simulink model "nonLinearSim"  (R2021b)
settings: Solver=VariableStepAuto  StartTime=0.0  StopTime=50  MaxStep=0.01  RelTol=1e-3
undefined symbols (not defined in the file or in its folder): IRL, P, PE, SE
settings Model: Creator=rushik  LastModifiedBy=rushik
settings DataIOCC: SaveOutput=off  DSMLogging=off  SaveTime=off  ReturnWorkspaceOutputs=off

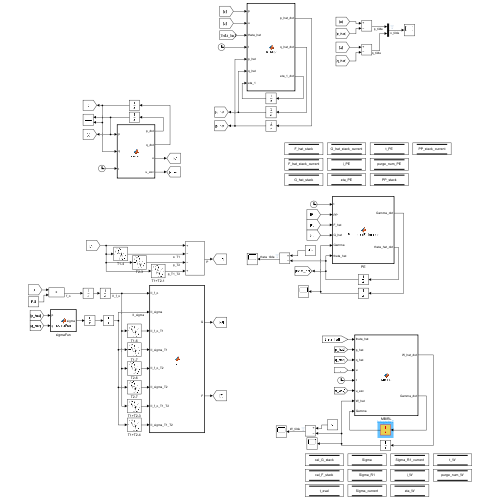
[thumbnail: Simulink's stored preview of the top-level diagram]
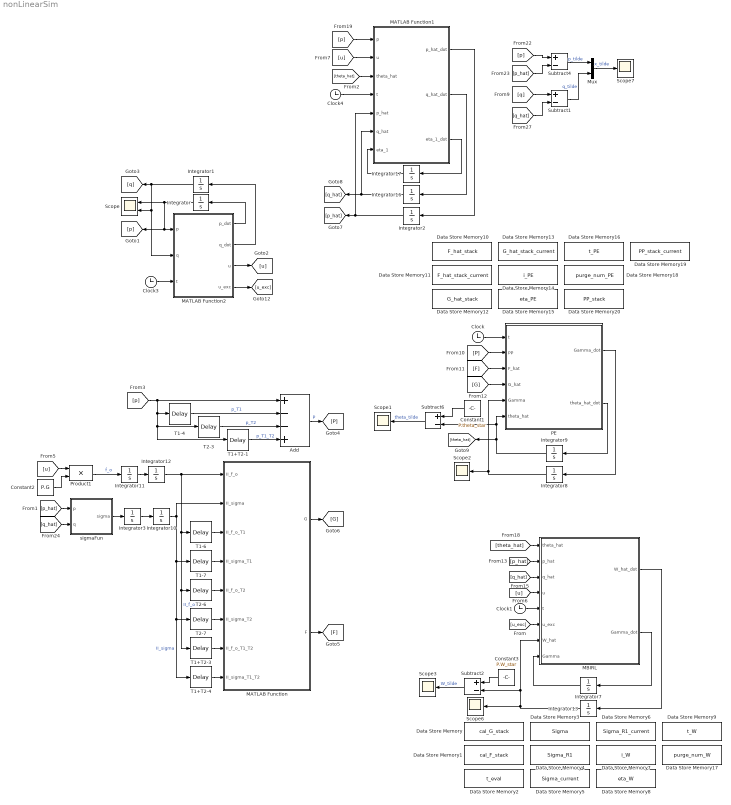
== system nonLinearSim ==
  Add : Sum  Inputs=+--+
  Clock{,1,3..4} (4 alike) : Clock
  Constant1 : Constant  Value=P.theta_star
  Constant2 : Constant  Value=P.G
  Constant3 : Constant  Value=P.W_star  VectorParams1D=off
  Data Store Memory : DataStoreMemory  DataStoreName=cal_G_stack  ReadBeforeWriteMsg=warning  WriteAfterWriteMsg=warning  WriteAfterReadMsg=warning  InitialValue=zeros(2*P.n^2,P.n*PE.N)  VectorParams1D=off  ShowAdditionalParam=off  OutDataTypeStr=double
  Data Store Memory1 : DataStoreMemory  DataStoreName=cal_F_stack  ReadBeforeWriteMsg=warning  WriteAfterWriteMsg=warning  WriteAfterReadMsg=warning  InitialValue=zeros(P.n,PE.N)  VectorParams1D=off  ShowAdditionalParam=off  OutDataTypeStr=double
  Data Store Memory10 : DataStoreMemory  DataStoreName=F_hat_stack  ReadBeforeWriteMsg=warning  WriteAfterWriteMsg=warning  WriteAfterReadMsg=warning  InitialValue=zeros(P.n,PE.N)  VectorParams1D=off  ShowAdditionalParam=off  OutDataTypeStr=double
  Data Store Memory11 : DataStoreMemory  DataStoreName=F_hat_stack_current  ReadBeforeWriteMsg=warning  WriteAfterWriteMsg=warning  WriteAfterReadMsg=warning  InitialValue=zeros(P.n,PE.N)  VectorParams1D=off  ShowAdditionalParam=off  OutDataTypeStr=double
  Data Store Memory12 : DataStoreMemory  DataStoreName=G_hat_stack  ReadBeforeWriteMsg=warning  WriteAfterWriteMsg=warning  WriteAfterReadMsg=warning  InitialValue=zeros(PE.L,PE.N)  VectorParams1D=off  ShowAdditionalParam=off  OutDataTypeStr=double
  Data Store Memory13 : DataStoreMemory  DataStoreName=G_hat_stack_current  ReadBeforeWriteMsg=warning  WriteAfterWriteMsg=warning  WriteAfterReadMsg=warning  InitialValue=zeros(PE.L,PE.N)  VectorParams1D=off  ShowAdditionalParam=off  OutDataTypeStr=double
  Data Store Memory14 : DataStoreMemory  DataStoreName=i_PE  ReadBeforeWriteMsg=warning  WriteAfterWriteMsg=warning  WriteAfterReadMsg=warning  InitialValue=1  VectorParams1D=off  ShowAdditionalParam=off  OutDataTypeStr=double
  Data Store Memory15 : DataStoreMemory  DataStoreName=eta_PE  ReadBeforeWriteMsg=warning  WriteAfterWriteMsg=warning  WriteAfterReadMsg=warning  VectorParams1D=off  ShowAdditionalParam=off  OutDataTypeStr=double
  Data Store Memory16 : DataStoreMemory  DataStoreName=t_PE  ReadBeforeWriteMsg=warning  WriteAfterWriteMsg=warning  WriteAfterReadMsg=warning  VectorParams1D=off  ShowAdditionalParam=off  OutDataTypeStr=double
  Data Store Memory17 : DataStoreMemory  DataStoreName=purge_num_W  ReadBeforeWriteMsg=warning  WriteAfterWriteMsg=warning  WriteAfterReadMsg=warning  VectorParams1D=off  ShowAdditionalParam=off  OutDataTypeStr=double
  Data Store Memory18 : DataStoreMemory  DataStoreName=purge_num_PE  ReadBeforeWriteMsg=warning  WriteAfterWriteMsg=warning  WriteAfterReadMsg=warning  VectorParams1D=off  ShowAdditionalParam=off  OutDataTypeStr=double
  Data Store Memory19 : DataStoreMemory  DataStoreName=PP_stack_current  ReadBeforeWriteMsg=warning  WriteAfterWriteMsg=warning  WriteAfterReadMsg=warning  InitialValue=zeros(P.n,PE.N)  VectorParams1D=off  ShowAdditionalParam=off  OutDataTypeStr=double
  Data Store Memory2 : DataStoreMemory  DataStoreName=t_eval  ReadBeforeWriteMsg=warning  WriteAfterWriteMsg=warning  WriteAfterReadMsg=warning  VectorParams1D=off  ShowAdditionalParam=off  OutDataTypeStr=double
  Data Store Memory20 : DataStoreMemory  DataStoreName=PP_stack  ReadBeforeWriteMsg=warning  WriteAfterWriteMsg=warning  WriteAfterReadMsg=warning  InitialValue=zeros(P.n,PE.N)  VectorParams1D=off  ShowAdditionalParam=off  OutDataTypeStr=double
  Data Store Memory3 : DataStoreMemory  DataStoreName=Sigma  ReadBeforeWriteMsg=warning  WriteAfterWriteMsg=warning  WriteAfterReadMsg=warning  InitialValue=zeros(2*IRL.N,IRL.num_weights)  VectorParams1D=off  ShowAdditionalParam=off  OutDataTypeStr=double
  Data Store Memory4 : DataStoreMemory  DataStoreName=Sigma_R1  ReadBeforeWriteMsg=warning  WriteAfterWriteMsg=warning  WriteAfterReadMsg=warning  InitialValue=zeros(2*IRL.N,1)  VectorParams1D=off  ShowAdditionalParam=off  OutDataTypeStr=double
  Data Store Memory5 : DataStoreMemory  DataStoreName=Sigma_current  ReadBeforeWriteMsg=warning  WriteAfterWriteMsg=warning  WriteAfterReadMsg=warning  InitialValue=zeros(2*IRL.N,IRL.num_weights)  VectorParams1D=off  ShowAdditionalParam=off  OutDataTypeStr=double
  Data Store Memory6 : DataStoreMemory  DataStoreName=Sigma_R1_current  ReadBeforeWriteMsg=warning  WriteAfterWriteMsg=warning  WriteAfterReadMsg=warning  InitialValue=zeros(2*IRL.N,1)  VectorParams1D=off  ShowAdditionalParam=off  OutDataTypeStr=double
  Data Store Memory7 : DataStoreMemory  DataStoreName=i_W  ReadBeforeWriteMsg=warning  WriteAfterWriteMsg=warning  WriteAfterReadMsg=warning  InitialValue=1  VectorParams1D=off  ShowAdditionalParam=off  OutDataTypeStr=double
  Data Store Memory8 : DataStoreMemory  DataStoreName=eta_W  ReadBeforeWriteMsg=warning  WriteAfterWriteMsg=warning  WriteAfterReadMsg=warning  VectorParams1D=off  ShowAdditionalParam=off  OutDataTypeStr=double
  Data Store Memory9 : DataStoreMemory  DataStoreName=t_W  ReadBeforeWriteMsg=warning  WriteAfterWriteMsg=warning  WriteAfterReadMsg=warning  VectorParams1D=off  ShowAdditionalParam=off  OutDataTypeStr=double
  Integrator : Integrator  InitialCondition=P.p_0
  Integrator1 : Integrator  InitialCondition=P.q_0
  Integrator10 : Integrator  InitialCondition=zeros(PE.L,1)
  Integrator11 : Integrator  InitialCondition=zeros(P.n,1)
  Integrator12 : Integrator  InitialCondition=zeros(P.n,1)
  Integrator13 : Integrator  InitialCondition=IRL.W_hat_0
  Integrator16 : Integrator  InitialCondition=SE.q_hat_0
  Integrator17 : Integrator
  Integrator2 : Integrator  InitialCondition=P.p_0
  Integrator3 : Integrator  InitialCondition=zeros(PE.L,1)
  Integrator7 : Integrator  InitialCondition=IRL.Gamma_W_0
  Integrator8 : Integrator  InitialCondition=PE.Gamma_0
  Integrator9 : Integrator  InitialCondition=PE.theta_hat_0
  MATLAB Function : MATLAB Function  TreatAsAtomicUnit=on
  MATLAB Function1 : MATLAB Function  TreatAsAtomicUnit=on
  MATLAB Function2 : MATLAB Function  TreatAsAtomicUnit=on
  MBIRL : MATLAB Function  TreatAsAtomicUnit=on
  Mux : Mux  Inputs=2
  PE : MATLAB Function  TreatAsAtomicUnit=on
  Product1 : Product
  Scope : Scope  NumInputPorts=2
  Scope{1..3,6..7} (5 alike) : Scope
  Subtract{1..2,4,6} (4 alike) : Sum  Inputs=+-
  T1+T2-1 : TransportDelay  DelayTime=PE.T2 + PE.T1
  T1+T2-3 : TransportDelay  DelayTime=PE.T2 + PE.T1
  T1+T2-4 : TransportDelay  DelayTime=PE.T2 + PE.T1
  T1-4 : TransportDelay  DelayTime=PE.T1
  T1-6 : TransportDelay  DelayTime=PE.T1
  T1-7 : TransportDelay  DelayTime=PE.T1
  T2-3 : TransportDelay  DelayTime=PE.T2
  T2-6 : TransportDelay  DelayTime=PE.T2
  T2-7 : TransportDelay  DelayTime=PE.T2
  sigmaFun : MATLAB Function  TreatAsAtomicUnit=on
  wires:
  MATLAB Function2/1(p_dot) -> Integrator/1
  MATLAB Function2/2(q_dot) -> Integrator1/1
  Integrator1/1 -> [q], MATLAB Function2/2(q), Scope/2
  MATLAB Function2/3(u) -> [u]
  Integrator3/1 -> Integrator10/1
  Integrator/1 -> Scope/1, [p], MATLAB Function2/1(p)
  T1-4/1 -> Add/2  "p_T1"
  T2-3/1 -> Add/3  "p_T2"
  T1+T2-1/1 -> Add/4  "p_T1_T2"
  PE/1(Gamma_dot) -> Integrator8/1
  Clock/1 -> PE/1(t)
  Integrator8/1 -> Scope2/1, PE/5(Gamma)
  PE/2(theta_hat_dot) -> Integrator9/1
  Integrator9/1 -> [theta_hat], PE/6(theta_hat), Subtract6/2
  Constant1/1 -> Subtract6/1
  Subtract6/1 -> Scope1/1  "theta_tilde"
  Constant2/1 -> Product1/2
  Product1/1 -> Integrator11/1  "f_o"
  Integrator11/1 -> Integrator12/1
  T1-6/1 -> MATLAB Function/3(II_f_o_T1)
  T1-7/1 -> MATLAB Function/4(II_sigma_T1)
  T2-6/1 -> MATLAB Function/5(II_f_o_T2)
  T1+T2-3/1 -> MATLAB Function/7(II_f_o_T1_T2)
  MATLAB Function/2(F) -> [F]
  Subtract1/1 -> Mux/2  "q_tilde"
  MBIRL/2(Gamma_dot) -> Integrator7/1
  Integrator7/1 -> MBIRL/8(Gamma)
  MBIRL/1(W_hat_dot) -> Integrator13/1
  Integrator13/1 -> Scope6/1, MBIRL/7(W_hat), Subtract2/2
  Subtract2/1 -> Scope3/1  "W_tilde"
  Constant3/1 -> Subtract2/1
  [p_hat] -> sigmaFun/1(p)
  [p] -> T1+T2-1/1, T2-3/1, T1-4/1, Add/1
  [u] -> Product1/1
  [u] -> MBIRL/4(u)
  [q] -> Subtract1/1
  [F] -> PE/3(F_hat)
  MATLAB Function/1(G) -> [G]
  [G] -> PE/4(G_hat)
  Clock1/1 -> MBIRL/5(t)
  [p_hat] -> MBIRL/2(p_hat)
  [q_hat] -> MBIRL/3(q_hat)
  [theta_hat] -> MBIRL/1(theta_hat)
  [p] -> Subtract4/1
  [p_hat] -> Subtract4/2
  Subtract4/1 -> Mux/1  "p_tilde"
  Mux/1 -> Scope7/1  "x_tilde"
  MATLAB Function2/4(u_exc) -> [u_exc]
  Clock3/1 -> MATLAB Function2/3(t)
  Integrator12/1 -> T1+T2-3/1, T2-6/1, T1-6/1, MATLAB Function/1(II_f_o)  "II_f_o"
  Integrator10/1 -> T1+T2-4/1, T2-7/1, T1-7/1, MATLAB Function/2(II_sigma)  "II_sigma"
  [q_hat] -> sigmaFun/2(q)
  T2-7/1 -> MATLAB Function/6(II_sigma_T2)
  T1+T2-4/1 -> MATLAB Function/8(II_sigma_T1_T2)
  Add/1 -> [P]  "P"
  [P] -> PE/2(PP)
  sigmaFun/1(sigma) -> Integrator3/1
  [q_hat] -> Subtract1/2
  MATLAB Function1/3(eta_1_dot) -> Integrator17/1
  Integrator17/1 -> MATLAB Function1/7(eta_1)
  MATLAB Function1/2(q_hat_dot) -> Integrator16/1
  Integrator16/1 -> [q_hat], MATLAB Function1/6(q_hat)
  MATLAB Function1/1(p_hat_dot) -> Integrator2/1
  Integrator2/1 -> [p_hat], MATLAB Function1/5(p_hat)
  [u] -> MATLAB Function1/2(u)
  [p] -> MATLAB Function1/1(p)
  Clock4/1 -> MATLAB Function1/4(t)
  [theta_hat] -> MATLAB Function1/3(theta_hat)
  [u_exc] -> MBIRL/6(u_exc)

== matlab function nonLinearSim/sigmaFun ==
  data: p input; sigma output; q input
function sigma = sigmaFun(p,q)
    sigma = [p*(pi/2+atan(5*p)); p^2/(1+25*p^2); q];
end

== matlab function nonLinearSim/MATLAB Function1 ==
  data: p input; u input; theta_hat input; t input; p_hat input; q_hat input; eta_1 input; p_hat_dot output; q_hat_dot output; eta_1_dot output; P parameter; SE parameter
function [p_hat_dot,q_hat_dot,eta_1_dot] = R_filter(p,u,theta_hat,t,p_hat,q_hat,eta_1,P, SE)
    p_tilde = p - p_hat;
    Y_hat = [p_hat*(pi/2+atan(5*p_hat)), p_hat*p_hat/(1+25*p_hat*p_hat), q_hat];
    p_hat_dot = q_hat;
    q_hat_dot = Y_hat*theta_hat + P.G*u + SE.alpha^2*p_tilde - (SE.k+SE.alpha+SE.beta)*eta_1 + (SE.k+SE.alpha)*(SE.k+SE.alpha+SE.beta)*p_tilde;
    eta_1_dot = -(SE.k+SE.beta)*eta_1 + ((SE.k+SE.beta)*(SE.k+SE.alpha)-SE.k*SE.alpha)*p_tilde;
end

== matlab function nonLinearSim/PE ==
  settings: updateMethod=DISCRETE
  data: t input; Gamma_dot output; PP input; F_hat input; G_hat input; Gamma input; theta_hat input; theta_hat_dot output; P parameter; PE parameter; G_hat_stack data_store_memory; F_hat_stack data_store_memory; t_PE data_store_memory; F_hat_stack_current data_store_memory; G_hat_stack_current data_store_memory; PP_stack_current data_store_memory; PP_stack data_store_memory; purge_num_PE data_store_memory; i_PE data_store_memory; eta_PE data_store_memory
function [Gamma_dot,theta_hat_dot]  = ParameterEstimation(t,PP,F_hat,G_hat,Gamma,theta_hat,P,PE)
    %#codegen
    
    global F_hat_stack G_hat_stack PP_stack
    global F_hat_stack_current
    global G_hat_stack_current PP_stack_current
    global t_PE eta_PE i_PE purge_num_PE
    
    if purge_num_PE == 0
        theta_hat_dot = zeros(PE.L,P.n);
        Gamma_dot = zeros(PE.L);
    else
        theta_hat_dot = PE.k_theta*Gamma*(G_hat_stack_current*...
            (PP_stack_current.' - F_hat_stack_current.'...
            - G_hat_stack_current.'*theta_hat));
            
        Gamma_dot = PE.beta*Gamma - PE.k_theta*Gamma*...
            (G_hat_stack_current*G_hat_stack_current.')*Gamma;
    end
    if t - t_PE >= PE.t_step && t >= PE.T1 + PE.T2
        if i_PE <= PE.N
            G_hat_stack(:,i_PE) = G_hat;
            F_hat_stack(:,i_PE) = F_hat;
            PP_stack(:,i_PE) = PP;
            i_PE = i_PE + 1;
            eta_PE = t;
        else
            new_script_G = G_hat_stack*G_hat_stack.';
            new_singular_value = min(svd(new_script_G));
            singular_value_list = zeros(PE.N,1);
            for i=1:PE.N
                ith_G_hat = G_hat_stack(:,i);
                new_script_G = new_script_G + G_hat*G_hat.'...
                    -ith_G_hat*ith_G_hat.';
                singular_value_list(i,1)=min(svd(new_script_G));
            end
            [singular_value_after_rep,max_index]=max(singular_value_list);
            
            if singular_value_after_rep >= new_singular_value
                G_hat_stack(:,max_index) = G_hat;
                F_hat_stack(:,max_index) = F_hat;
                PP_stack(:,max_index) = PP;
                new_singular_value = singular_value_after_rep;
            end
            if new_singular_value > 1e-10
                G_hat_stack_current = G_hat_stack;
                F_hat_stack_current = F_hat_stack;
                PP_stack_current = PP_stack;
                if abs(eta_PE-t) > PE.tau  
                    G_hat_stack_current = G_hat_stack;
                    F_hat_stack_current = F_hat_stack;
                    PP_stack_current = PP_stack;
                    i_PE=1;
                    eta_PE=t;
                    purge_num_PE = purge_num_PE + 1;
                end
            end
        end
        t_PE = t;  
    end
end

== matlab function nonLinearSim/MATLAB Function ==
  data: II_f_o input; G output; II_sigma input; II_f_o_T1 input; F output; II_sigma_T1 input; II_f_o_T2 input; II_sigma_T2 input; II_f_o_T1_T2 input; II_sigma_T1_T2 input
function [G, F] = generateIntegrals(II_f_o,II_sigma,II_f_o_T1,II_sigma_T1,II_f_o_T2,II_sigma_T2,II_f_o_T1_T2,II_sigma_T1_T2)

F = II_f_o - II_f_o_T1 - II_f_o_T2 + II_f_o_T1_T2;

G = II_sigma - II_sigma_T1 - II_sigma_T2 + II_sigma_T1_T2;

end

== matlab function nonLinearSim/MATLAB Function2 ==
  data: p input; p_dot output; q input; t input; q_dot output; P parameter; u output; u_exc output
function [p_dot,q_dot,u,u_exc] = system(p,q,t,P)
    %P.theta_star = [-1;-5/2;4];
    p_dot=q;
    Y = [p*(pi/2+atan(5*p)), p*p/(1+25*p*p), q];
    u_star = -3*q;
    u_exc = 9*cos(3*t) + 6*cos(2*t) + 3*cos(t)+ 15*cos(5*t);
    u = u_star + u_exc;
    q_dot=Y*P.theta_star + P.G*u;
end

== matlab function nonLinearSim/MBIRL ==
  settings: updateMethod=DISCRETE
  data: theta_hat input; p_hat input; q_hat input; u input; t input; u_exc input; W_hat input; P parameter; W_hat_dot output; Gamma_dot output; IRL parameter; t_W data_store_memory; Sigma data_store_memory; Sigma_R1 data_store_memory; Sigma_R1_current data_store_memory; Sigma_current data_store_memory; i_W data_store_memory; eta_W data_store_memory; Gamma input; purge_num_W data_store_memory; PE parameter
function [W_hat_dot,Gamma_dot] = MBIRL(theta_hat,p_hat,q_hat,u,t,u_exc,W_hat,P,IRL,Gamma,PE)

global Sigma Sigma_R1 Sigma_current Sigma_R1_current i_W eta_W t_W purge_num_W

mu = u - u_exc;

grad_x_sigma_V= [[ 2*p_hat,                                                0      ];
                 [ 2*p_hat*atan(5*p_hat)+5*p_hat*p_hat/(25*p_hat*p_hat+1), 0      ];
                 [ 0,                                                      2*q_hat]];

IRL_theta_hat = [zeros(size(theta_hat)), theta_hat];
sigma_hat = [p_hat*(pi/2+atan(5*p_hat)); p_hat^2/(1+25*p_hat^2); q_hat];

f_o = [q_hat; zeros(size(q_hat))] + [zeros(P.n,1);P.G]*mu;
Y_hat = f_o + IRL_theta_hat.'*sigma_hat;

sigma_Q_hat = [p_hat^2;q_hat^2];
sigma_R1_minus = [];
sigma_double_prime = [grad_x_sigma_V*Y_hat;sigma_Q_hat;sigma_R1_minus];

grad_u_f_o = [zeros(P.n,1);P.G];
grad_u_sigma = zeros(size(sigma_hat));
G = grad_u_f_o.'*grad_x_sigma_V.' + (IRL_theta_hat.'*grad_u_sigma).'*grad_x_sigma_V.';
sigma_R2_minus = [];
sigma_triple_prime = [sigma_double_prime [G.';zeros(numel(sigma_Q_hat),P.m);2*sigma_R2_minus.']];
sigma_R1 = [P.R(1,1)*mu^2;2*P.R(1,1)*mu];

if purge_num_W == 0
    W_hat_dot = zeros(IRL.num_weights,1);
    Gamma_dot = zeros(IRL.num_weights,IRL.num_weights);
else
    W_hat_dot = IRL.alpha*Gamma*Sigma_current'*(-Sigma_current*W_hat+Sigma_R1_current);
    Gamma_dot = IRL.beta*Gamma - IRL.alpha*Gamma*(Sigma_current'*Sigma_current)*Gamma;
end

if t - t_W >= IRL.t_step
    if i_W <= IRL.N
        Sigma(2*i_W-1:2*i_W,:) = sigma_triple_prime.';
        Sigma_R1(2*i_W-1:2*i_W,:) = -sigma_R1;
        i_W = i_W + 1;
        eta_W = t;
    else
        new_SST = Sigma.'*Sigma;
        new_con_num = cond(new_SST);
        con_num_list = zeros(IRL.N,1);
        for i=1:IRL.N
            ith_sigma = Sigma(2*i-1:2*i,:);
            new_SST = new_SST + sigma_triple_prime*sigma_triple_prime.'...
                -ith_sigma.'*ith_sigma;
            con_num_list(i,1)=cond(new_SST);
        end
        [c_num_aft_rep,ind]=min(con_num_list);
        if c_num_aft_rep < new_con_num
            Sigma(2*ind-1:2*ind,:) = sigma_triple_prime.';
            Sigma_R1(2*ind-1:2*ind,:) = -sigma_R1;
            new_con_num = c_num_aft_rep;
        end
        if new_con_num < 1e20
            Sigma_current = Sigma;
            Sigma_R1_current = Sigma_R1;
            if abs(eta_W-t) > IRL.tau
               Sigma = zeros(2*IRL.N,IRL.num_weights);
               Sigma_R1 = zeros(2*IRL.N,1);
               i_W=1;
               eta_W=t;
               purge_num_W = purge_num_W + 1;
            end
        end
    end
    t_W = t;
end
end
